simulink model "Sim_IsoSysOf4F"  (R2016b)
settings: Solver=FixedStepAuto  StartTime=0.0  StopTime=Tsim  FixedStep=0.01  RelTol=1e-3
values from neighbouring files (symbols this model uses):
  A = X(:,8)    [IsoSysOf4F.m]
  As = [zeros(3,3),eye(3,3) ... (first row only)    [StructModel_BLWN.m]
  Bs = [zeros(3,1) ... (first row only)    [StructModel_BLWN.m]
  Cs = [eye(DoF)+diag(-ones(DoF-1,1),-1),zeros(DoF)]    [StructModel_BLWN.m]
  Ds = zeros(DoF,1)    [StructModel_BLWN.m]
  T = X(:,7)    [IsoSysOf4F.m]
settings Model: Creator=dsmj  LastModifiedBy=dsmj

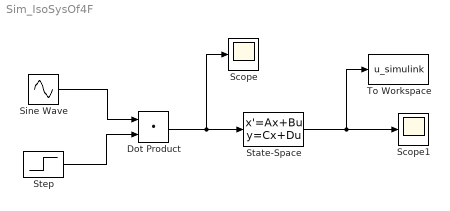
== system Sim_IsoSysOf4F ==
  Dot Product : DotProduct  InputSameDT=on  OutDataTypeStr=Inherit: Inherit via internal rule
  Scope : Scope
  Scope1 : Scope
  Sine Wave : Sin  Amplitude=A  Frequency=2*pi/T  SampleTime=0
  State-Space : StateSpace  A=As  B=Bs  C=Cs  D=Ds  X0=0
  Step : Step  Time=T  Before=1  After=0  SampleTime=0
  To Workspace : ToWorkspace  VariableName=u_simulink  SaveFormat=Timeseries  SampleTime=-1
  wires:
  State-Space/1 -> To Workspace/1, Scope1/1
  Step/1 -> Dot Product/2
  Sine Wave/1 -> Dot Product/1
  Dot Product/1 -> Scope/1, State-Space/1
